simulink model "HillyCond_SIL"  (R2021a)
settings: Solver=FixedStepDiscrete  StartTime=0.0  StopTime=10.0  FixedStep=0.01  RelTol=1e-3
libraries: pil_lib x1
settings Model: Creator=hp  LastModifiedBy=hp
settings OptimizationCC: DefaultParameterBehavior=Inlined  EnhancedBackFolding=on  PassReuseOutputArgsAs=Individual arguments  ZeroExternalMemoryAtStartup=off  ZeroInternalMemoryAtStartup=off  InitFltsAndDblsToZero=on  OptimizeBlockOrder=speed  DifferentSizesBufferReuse=on  OptimizationCustomize=off  EfficientTunableParamExpr=on
settings DebuggingCC: SignalInfNanChecking=error  CheckMatrixSingularityMsg=error  IntegerOverflowMsg=error  ParameterTunabilityLossMsg=error  UnderSpecifiedDataTypeMsg=warning  UniqueDataStoreMsg=warning  StrictBusMsg=ErrorOnBusTreatedAsVector  IntegerSaturationMsg=error
settings HardwareCC: TargetLongLongMode=on
settings SFSimCC: MATLABDynamicMemAlloc=off
settings RTWCC: SystemTargetFile=ert.tlc  TemplateMakefile=ert_default_tmf  GenerateReport=on  Toolchain=MinGW64 | gmake (64-bit Windows)  IncludeHyperlinkInReport=on  LaunchReport=on  GenerateTraceInfo=on  GenerateTraceReport=on  GenerateTraceReportSl=on  GenerateTraceReportSf=on
settings CodeAppCC: ForceParamTrailComments=on  IgnoreCustomStorageClasses=off  OperatorAnnotations=on  SimulinkDataObjDesc=on  SFDataObjDesc=on  InsertBlockDesc=on
settings ERTTargetCC: TargetLangStandard=C99 (ISO)  GenerateSampleERTMain=on  InlinedParameterPlacement=NonHierarchical  ERTCustomFileTemplate=example_file_process.tlc

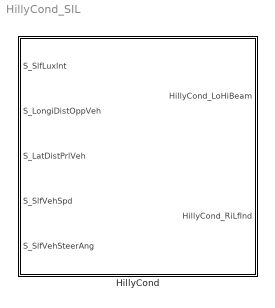
== system HillyCond_SIL ==
  HillyCond : Subsystem  DialogController=pil_create_dialog  LoadFcn=|  TreatAsAtomicUnit=on
      | try
      |    if ~strcmp(rtw.pil.getPILVersion, '9.10 (R2021a)_15')
      |       set_param(gcb, 'DialogController', '');
      |       set_param(gcb, 'DialogControllerArgs', '');
      |    end
      | catch e
      |       set_param(gcb, 'DialogController', '');
      |       set_param(gcb, 'DialogControllerArgs', '');
      | end
      mask help: PIL:pil:XILBlockMaskDesc
      mask Display: disp('SIL');

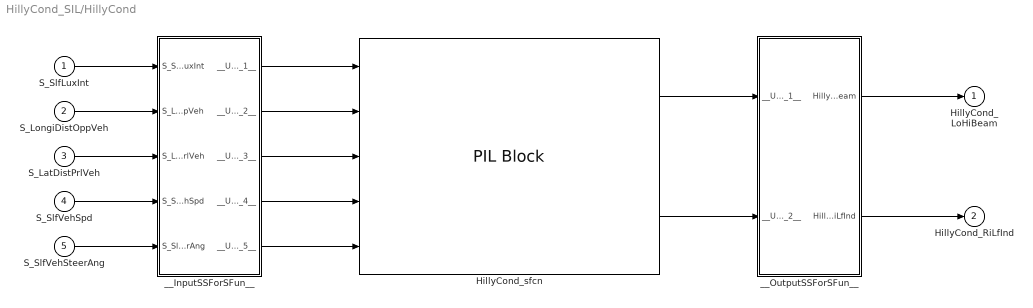
== system HillyCond_SIL/HillyCond ==
  S_SlfLuxInt : Inport
  S_LongiDistOppVeh : Inport  Port=2
  S_LatDistPrlVeh : Inport  Port=3
  S_SlfVehSpd : Inport  Port=4
  S_SlfVehSteerAng : Inport  Port=5
  HillyCond_sfcn : pil_lib/PIL Block  SimulationMode=SIL  IsTopModelPIL=off  CodeDir=C:\Adaptive_Front_Light_System_V1.0.0\AFLS_V1.0.0\ASW\SWC\Hilly\Mdl\HillyCond_ert_rtw  AnchorDir=C:\Adaptive_Front_Light_System_V1.0.0\AFLS_V1.0.0\ASW\SWC\Hilly\Mdl  ConfigName=Software-in-the-Loop (SIL)  XrelIsTopModelCode=on  XrelIsReusable=off  XrelDWorkNames={}  XrelDWorkTypes={}  XrelModelArgVals={}  XrelOrderedParamNames={}
      settings: SourceProductBaseCode=RT
  __InputSSForSFun__ : Subsystem
  __OutputSSForSFun__ : Subsystem
  HillyCond_LoHiBeam : Outport
  HillyCond_RiLfInd : Outport  Port=2
  wires:
  S_SlfLuxInt/1 -> __InputSSForSFun__/1(S_SlfLuxInt)
  S_LongiDistOppVeh/1 -> __InputSSForSFun__/2(S_LongiDistOppVeh)
  S_LatDistPrlVeh/1 -> __InputSSForSFun__/3(S_LatDistPrlVeh)
  S_SlfVehSpd/1 -> __InputSSForSFun__/4(S_SlfVehSpd)
  S_SlfVehSteerAng/1 -> __InputSSForSFun__/5(S_SlfVehSteerAng)
  __InputSSForSFun__/1(__UniqueOutportName__1__) -> HillyCond_sfcn/1
  __InputSSForSFun__/2(__UniqueOutportName__2__) -> HillyCond_sfcn/2
  __InputSSForSFun__/3(__UniqueOutportName__3__) -> HillyCond_sfcn/3
  __InputSSForSFun__/4(__UniqueOutportName__4__) -> HillyCond_sfcn/4
  __InputSSForSFun__/5(__UniqueOutportName__5__) -> HillyCond_sfcn/5
  HillyCond_sfcn/1 -> __OutputSSForSFun__/1(__UniqueInportName__1__)
  HillyCond_sfcn/2 -> __OutputSSForSFun__/2(__UniqueInportName__2__)
  __OutputSSForSFun__/1(HillyCond_LoHiBeam) -> HillyCond_LoHiBeam/1
  __OutputSSForSFun__/2(HillyCond_RiLfInd) -> HillyCond_RiLfInd/1

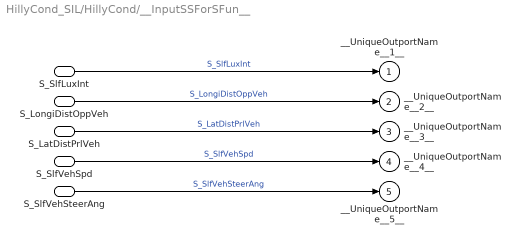
== system HillyCond_SIL/HillyCond/__InputSSForSFun__ ==
  S_SlfLuxInt : Inport
  S_LongiDistOppVeh : Inport  Port=2
  S_LatDistPrlVeh : Inport  Port=3
  S_SlfVehSpd : Inport  Port=4
  S_SlfVehSteerAng : Inport  Port=5
  __UniqueOutportName__1__ : Outport
  __UniqueOutportName__2__ : Outport  Port=2
  __UniqueOutportName__3__ : Outport  Port=3
  __UniqueOutportName__4__ : Outport  Port=4
  __UniqueOutportName__5__ : Outport  Port=5
  wires:
  S_SlfLuxInt/1 -> __UniqueOutportName__1__/1  "S_SlfLuxInt"
  S_LongiDistOppVeh/1 -> __UniqueOutportName__2__/1  "S_LongiDistOppVeh"
  S_LatDistPrlVeh/1 -> __UniqueOutportName__3__/1  "S_LatDistPrlVeh"
  S_SlfVehSpd/1 -> __UniqueOutportName__4__/1  "S_SlfVehSpd"
  S_SlfVehSteerAng/1 -> __UniqueOutportName__5__/1  "S_SlfVehSteerAng"

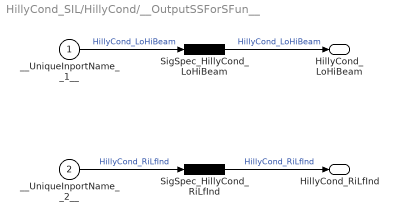
== system HillyCond_SIL/HillyCond/__OutputSSForSFun__ ==
  __UniqueInportName__1__ : Inport
  __UniqueInportName__2__ : Inport  Port=2
  SigSpec_HillyCond_LoHiBeam : Demux  Outputs=1
  SigSpec_HillyCond_RiLfInd : Demux  Outputs=1
  HillyCond_LoHiBeam : Outport
  HillyCond_RiLfInd : Outport  Port=2
  wires:
  __UniqueInportName__1__/1 -> SigSpec_HillyCond_LoHiBeam/1  "HillyCond_LoHiBeam"
  SigSpec_HillyCond_LoHiBeam/1 -> HillyCond_LoHiBeam/1  "HillyCond_LoHiBeam"
  __UniqueInportName__2__/1 -> SigSpec_HillyCond_RiLfInd/1  "HillyCond_RiLfInd"
  SigSpec_HillyCond_RiLfInd/1 -> HillyCond_RiLfInd/1  "HillyCond_RiLfInd"
